simulink model "AutoParking_Parallel_MPC_v2"  (R2021b)
settings: Solver=VariableStepAuto  StartTime=0  StopTime=25  FixedStep=0.01  RelTol=1e-3  AbsTol=1e-6
PreLoadFcn:
  | ParhPoint_Parallel
values from neighbouring files (symbols this model uses):
  dkappa_1 = [dkappa_1,dkappa_1(end)]    [ParhPoint_Parallel.m]    (also in ParhPoint_Parallel1.m)
  dkappa_2 = [dkappa_2,dkappa_2(end)]    [ParhPoint_Parallel.m]    (also in ParhPoint_Parallel1.m)
  dkappa_3 = [dkappa_3,dkappa_3(end)]    [ParhPoint_Parallel.m]    (also in ParhPoint_Parallel1.m)
  dx_1 = [7.49700000000000,7.48700000000000,7.47700000000000,7.46700000000000,7.45700000000000,7.44700000000000,7.43700000000000,7.42700000000000,7.41700000000000,7.40700000000000,7.39700000000000,7.38700000000000,7.37700000000000,7.36700000000000,7.35700000000000,7.34700000000000,7.33700000000000,7.32700000000000,7.31700000000000,7.30700000000000,7.29700000000000,7.28700000000000,7.27700000000000,7.267000 ...(+10617 chars)    [ParhPoint_Parallel1.m]
  dx_2 = xmr01'    [ParhPoint_Parallel.m]    (also in ParhPoint_Parallel1.m = [dx_1(end),1.12])
  dx_3 = [dx_2(end),dx_2(end)]    [ParhPoint_Parallel.m]    (also in ParhPoint_Parallel1.m)
  dy_1 = [1.10000132390871,1.10003103093403,1.10009720896582,1.10019908067609,1.10033587377205,1.10050682098400,1.10071116005326,1.10094813372010,1.10121698971167,1.10151698072983,1.10184736443921,1.10220740345502,1.10259636533104,1.10301352254745,1.10345815249885,1.10392953748209,1.10442696468426,1.10494972617060,1.10549711887234,1.10606844457472,1.10666300990486,1.10728012631967,1.10791911009379,1.108579 ...(+11295 chars)    [ParhPoint_Parallel1.m]
  dy_2 = ymr01'    [ParhPoint_Parallel.m]    (also in ParhPoint_Parallel1.m = [dy_1(end),-1])
  dy_3 = [dy_2(end),dy_2(end)]    [ParhPoint_Parallel.m]    (also in ParhPoint_Parallel1.m)
  dyaw_1 = 0    [ParhPoint_Parallel1.m]
  path_x = [dx_1,dx_2,dx_3]    [ParhPoint_Parallel.m]    (also in ParhPoint_Parallel1.m)
  path_y = [dy_1,dy_2,dy_3]    [ParhPoint_Parallel.m]    (also in ParhPoint_Parallel1.m)
undefined symbols (not defined in the file or in its folder): dyaw_2, dyaw_3
libraries: Solver_SF x1, simulink x1
settings Model: Creator=pmather  LastModifiedBy=Shu
settings SolverCC: AutoScaleAbsTol=off  AlgebraicLoopSolver=TrustRegion
settings DataIOCC: SaveFormat=Array  SignalLoggingSaveFormat=ModelDataLogs  ReturnWorkspaceOutputs=off
settings OptimizationCC: BlockReduction=off  BooleanDataType=off  InitFltsAndDblsToZero=on  LifeSpan=inf
settings DebuggingCC: SaveWithParameterizedLinksMsg=none  UnderspecifiedInitializationDetection=Classic  MergeDetectMultiDrivingBlocksExec=none  SignalResolutionControl=TryResolveAllWithWarning  MultiTaskDSMMsg=warning  MultiTaskCondExecSysMsg=none  SFExecutionAtInitializationDiag=none  SFMachineParentedDataDiag=warning  ArithmeticOperatorsInVariantConditions=warning
settings HardwareCC: ProdBitPerPointer=32  ProdBitPerSizeT=32  ProdBitPerPtrDiffT=32  ProdLargestAtomicFloat=None  ProdIntDivRoundTo=Undefined  ProdEndianess=Unspecified  ProdWordSize=32  ProdHWDeviceType=32-bit Generic  TargetUnknown=on
settings ModelReferenceCC: PropagateSignalLabelsOutOfModel=off
settings SFSimCC: CustomCodeUndefinedFunction=UseInterfaceOnly
settings RTWCC: TemplateMakefile=grt_vc.tmf
settings CodeAppCC: StateflowObjectComments=on
settings GRTTargetCC: TargetLangStandard=C89/C90 (ANSI)  CombineOutputUpdateFcns=off  GRTInterface=on
settings ConfigComp: CovMetricSettings=dw  CovSaveCumulativeToWorkspaceVar=on  CovSaveSingleToWorkspaceVar=on

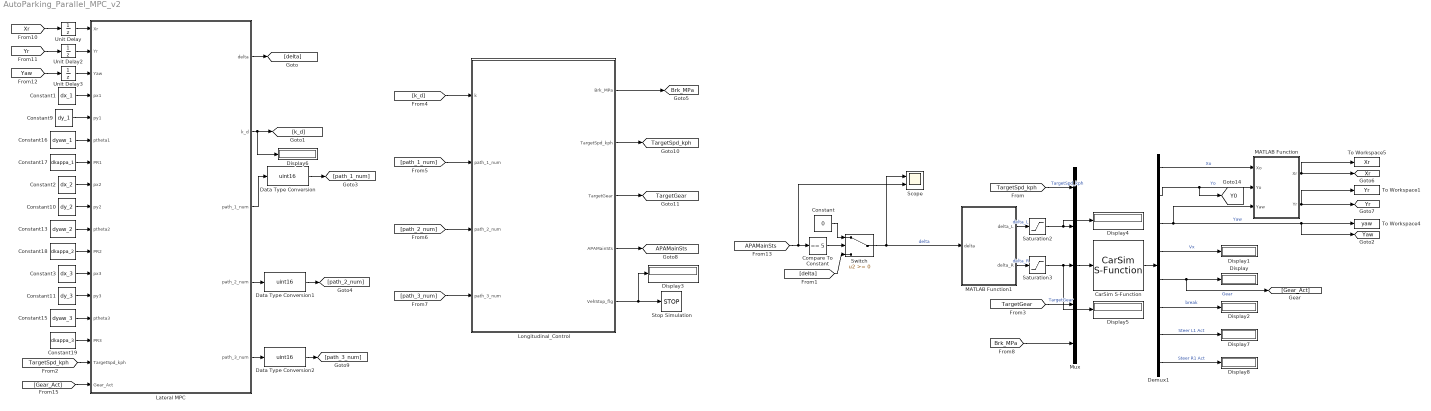
== system AutoParking_Parallel_MPC_v2 ==
  CarSim S-Function : Solver_SF/CarSim S-Function  Priority=1  SIMFILE=simfile.sim
  Compare To Constant : simulink/Logic and Bit Operations/Compare To Constant  relop===  const=5  OutDataTypeStr=boolean
  Constant : Constant  Value=0
  Constant1 : Constant  Value=dx_1
  Constant10 : Constant  Value=dy_2
  Constant11 : Constant  Value=dy_3
  Constant13 : Constant  Value=dyaw_2
  Constant15 : Constant  Value=dyaw_3
  Constant16 : Constant  Value=dyaw_1
  Constant17 : Constant  Value=dkappa_1
  Constant18 : Constant  Value=dkappa_2
  Constant19 : Constant  Value=dkappa_3
  Constant2 : Constant  Value=dx_2
  Constant3 : Constant  Value=dx_3
  Constant9 : Constant  Value=dy_1
  Data Type Conversion : DataTypeConversion  OutDataTypeStr=uint16
  Data Type Conversion1 : DataTypeConversion  OutDataTypeStr=uint16
  Data Type Conversion2 : DataTypeConversion  OutDataTypeStr=uint16
  Demux1 : Demux  Outputs=8
  Display{,1..8} (9 alike) : Display
  Lateral MPC : Subsystem
  Longitudinal_Control : Subsystem
  MATLAB Function : MATLAB Function  TreatAsAtomicUnit=on
  MATLAB Function1 : MATLAB Function  TreatAsAtomicUnit=on
  Mux : Mux  Inputs=5
  Saturation2 : Saturate  UpperLimit=34  LowerLimit=-34
  Saturation3 : Saturate  UpperLimit=34  LowerLimit=-34
  Scope : Scope  NumInputPorts=2
  Stop Simulation : Stop
  Switch : Switch
  To Workspace1 : ToWorkspace  VariableName=Yr  SaveFormat=Timeseries  SampleTime=-1
  To Workspace4 : ToWorkspace  VariableName=yaw  SaveFormat=Timeseries  SampleTime=-1
  To Workspace5 : ToWorkspace  VariableName=Xr  SaveFormat=Timeseries  SampleTime=-1
  Unit Delay : UnitDelay  InitialCondition=1.5  SampleTime=-1  HasFrameUpgradeWarning=on
  Unit Delay2 : UnitDelay  InitialCondition=2.5  SampleTime=-1  HasFrameUpgradeWarning=on
  Unit Delay3 : UnitDelay  SampleTime=-1  HasFrameUpgradeWarning=on
  tag scope: APAMainSts=global, Brk_MPa=global, TargetGear=global, TargetSpd_kph=global, Xr=global, Y0=global, Yaw=global, Yr=global
  wires:
  Mux/1 -> CarSim S-Function/1
  CarSim S-Function/1 -> Demux1/1
  Demux1/1 -> MATLAB Function/1(Xo)  "Xo"
  Demux1/2 -> [Y0], MATLAB Function/2(Yo)  "Yo"
  Demux1/3 -> [Yaw], To Workspace4/1, MATLAB Function/3(Yaw)  "Yaw"
  Demux1/4 -> Display1/1  "Vx"
  MATLAB Function/1(Xr) -> To Workspace5/1, [Xr]
  Longitudinal_Control/1(Brk_MPa) -> [Brk_MPa]
  [Yaw] -> Unit Delay3/1
  [Yr] -> Unit Delay2/1
  [Xr] -> Unit Delay/1
  Unit Delay2/1 -> Lateral MPC/2(Yr)
  Unit Delay/1 -> Lateral MPC/1(Xr)
  Unit Delay3/1 -> Lateral MPC/3(Yaw)
  Constant19/1 -> Lateral MPC/15(PR3)
  Constant18/1 -> Lateral MPC/11(PR2)
  Constant17/1 -> Lateral MPC/7(PR1)
  Constant15/1 -> Lateral MPC/14(ptheta3)
  Constant13/1 -> Lateral MPC/10(ptheta2)
  Constant16/1 -> Lateral MPC/6(ptheta1)
  Constant11/1 -> Lateral MPC/13(py3)
  Constant10/1 -> Lateral MPC/9(py2)
  Constant9/1 -> Lateral MPC/5(py1)
  Constant1/1 -> Lateral MPC/4(px1)
  Constant2/1 -> Lateral MPC/8(px2)
  Constant3/1 -> Lateral MPC/12(px3)
  [Brk_MPa] -> Mux/5
  Demux1/5 -> [Gear_Act], Display/1  "Gear"
  Demux1/6 -> Display2/1  "break"
  Longitudinal_Control/2(TargetSpd_kph) -> [TargetSpd_kph]
  [TargetSpd_kph] -> Mux/1  "TargetSpd_kph"
  Longitudinal_Control/3(TargetGear) -> [TargetGear]
  [TargetGear] -> Mux/4  "TargetGear"
  [TargetSpd_kph] -> Lateral MPC/16(TargetSpd_kph)
  MATLAB Function/2(Yr) -> To Workspace1/1, [Yr]
  Lateral MPC/1(delta) -> [delta]
  Lateral MPC/2(k_d) -> [k_d], Display6/1
  [k_d] -> Longitudinal_Control/1(k)
  [path_2_num] -> Longitudinal_Control/3(path_2_num)
  [path_3_num] -> Longitudinal_Control/4(path_3_num)
  [path_1_num] -> Longitudinal_Control/2(path_1_num)
  Lateral MPC/3(path_1_num) -> Data Type Conversion/1
  Data Type Conversion/1 -> [path_1_num]
  Lateral MPC/4(path_2_num) -> Data Type Conversion1/1
  Data Type Conversion1/1 -> [path_2_num]
  Lateral MPC/5(path_3_num) -> Data Type Conversion2/1
  Data Type Conversion2/1 -> [path_3_num]
  Demux1/7 -> Display7/1  "Steer L1 Act"
  Demux1/8 -> Display8/1  "Steer R1 Act"
  Saturation2/1 -> Display4/1, Mux/2
  Saturation3/1 -> Mux/3, Display5/1
  Longitudinal_Control/4(APAMainSts) -> [APAMainSts]
  Longitudinal_Control/5(VehStop_flg) -> Display3/1, Stop Simulation/1
  [Gear_Act] -> Lateral MPC/17(Gear_Act)
  Switch/1 -> MATLAB Function1/1(delta), Scope/1  "delta"
  MATLAB Function1/1(delta_L) -> Saturation2/1  "delta_L"
  MATLAB Function1/2(delta_R) -> Saturation3/1  "delta_R"
  [APAMainSts] -> Scope/2, Compare To Constant/1
  Compare To Constant/1 -> Switch/2
  Constant/1 -> Switch/1
  [delta] -> Switch/3

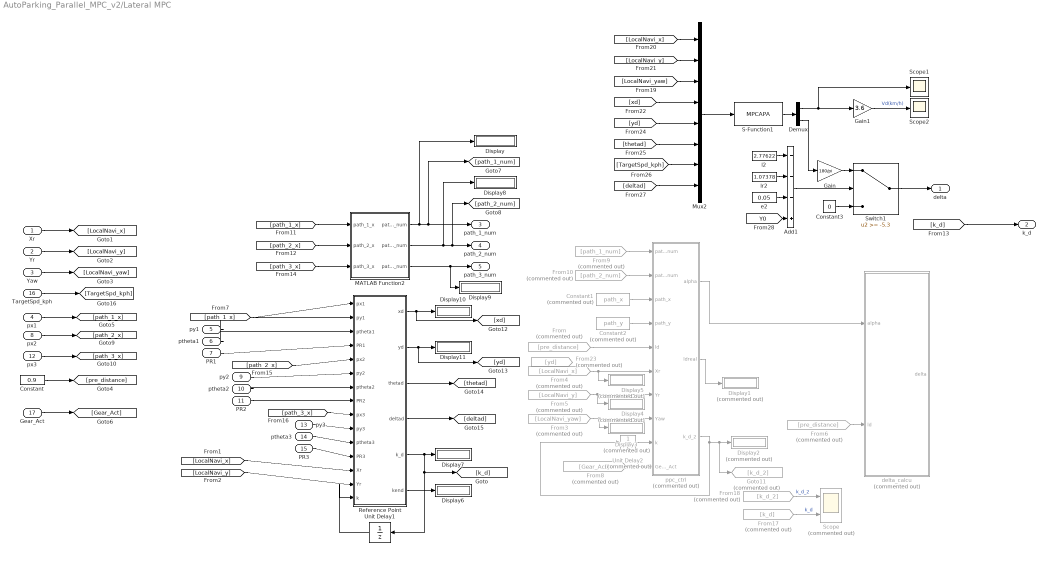
== system AutoParking_Parallel_MPC_v2/Lateral MPC ==
  Xr : Inport
  Yr : Inport  Port=2
  Yaw : Inport  Port=3
  px1 : Inport  Port=4
  py1 : Inport  Port=5
  ptheta1 : Inport  Port=6
  PR1 : Inport  Port=7
  px2 : Inport  Port=8
  py2 : Inport  Port=9
  ptheta2 : Inport  Port=10
  PR2 : Inport  Port=11
  px3 : Inport  Port=12
  py3 : Inport  Port=13
  ptheta3 : Inport  Port=14
  PR3 : Inport  Port=15
  TargetSpd_kph : Inport  Port=16
  Gear_Act : Inport  Port=17
  Add1 : Sum  Inputs=---+
  Constant : Constant  Value=0.9
  Constant1 : Constant  Commented=on  Value=path_x
  Constant2 : Constant  Commented=on  Value=path_y
  Constant3 : Constant  Value=0
  Demux : Demux  Outputs=2
  Display{,6..11} (7 alike) : Display
  Display{1..5} (5 alike) : Display  Commented=on
  From : From  Commented=on  GotoTag=pre_distance
  From10 : From  Commented=on  GotoTag=path_2_num
  From17 : From  Commented=on  GotoTag=k_d
  From18 : From  Commented=on  GotoTag=k_d_2
  From23 : From  Commented=on  GotoTag=yd
  From3 : From  Commented=on  GotoTag=LocalNavi_yaw
  From4 : From  Commented=on  GotoTag=LocalNavi_x
  From5 : From  Commented=on  GotoTag=LocalNavi_y
  From6 : From  Commented=on  GotoTag=pre_distance
  From8 : From  Commented=on  GotoTag=Gear_Act
  From9 : From  Commented=on  GotoTag=path_1_num
  Gain : Gain  Gain=180/pi
  Gain1 : Gain  Gain=3.6
  Goto11 : Goto  Commented=on  GotoTag=k_d_2
  MATLAB Function2 : MATLAB Function  TreatAsAtomicUnit=on
  Mux2 : Mux  Inputs=8
  Reference Point : MATLAB Function  TreatAsAtomicUnit=on
  S-Function1 : S-Function  FunctionName=MPCAPA  SFunctionDeploymentMode=off  EnableBusSupport=off
  Scope : Scope  Commented=on  NumInputPorts=2
  Scope1 : Scope
  Scope2 : Scope
  Switch1 : Switch  Threshold=-5.3
  Unit Delay1 : UnitDelay  InitialCondition=1  SampleTime=-1  HasFrameUpgradeWarning=on
  Unit Delay2 : UnitDelay  Commented=on  InitialCondition=1  SampleTime=-1  HasFrameUpgradeWarning=on
  delta_calcu : MATLAB Function  Commented=on  TreatAsAtomicUnit=on
  e2 : Constant  Value=0.05
  l2 : Constant  Value=2.77622
  lr2 : Constant  Value=1.07378
  ppc_ctrl : MATLAB Function  Commented=on  TreatAsAtomicUnit=on
  delta : Outport
  k_d : Outport  Port=2
  path_1_num : Outport  Port=3
  path_2_num : Outport  Port=4
  path_3_num : Outport  Port=5
  wires:
  Unit Delay1/1 -> Reference Point/15(k)
  Reference Point/5(k_d) -> Display7/1, [k_d], Unit Delay1/1
  py2/1 -> Reference Point/6(py2)
  ptheta2/1 -> Reference Point/7(ptheta2)
  PR2/1 -> Reference Point/8(PR2)
  py3/1 -> Reference Point/10(py3)
  ptheta3/1 -> Reference Point/11(ptheta3)
  PR3/1 -> Reference Point/12(PR3)
  Reference Point/3(thetad) -> [thetad]
  Reference Point/4(deltad) -> [deltad]
  TargetSpd_kph/1 -> [TargetSpd_kph]
  Xr/1 -> [LocalNavi_x]
  Yr/1 -> [LocalNavi_y]
  Yaw/1 -> [LocalNavi_yaw]
  [LocalNavi_x] -> Reference Point/13(Xr)
  [LocalNavi_y] -> Reference Point/14(Yr)
  Constant/1 -> [pre_distance]
  From/1 -> ppc_ctrl/5(ld)
  From5/1 -> Display4/1, ppc_ctrl/7(Yr)
  From4/1 -> Display5/1, ppc_ctrl/6(Xr)
  From3/1 -> Display3/1, ppc_ctrl/8(Yaw)
  ppc_ctrl/1(alpha) -> delta_calcu/1(alpha)
  ppc_ctrl/2(ldreal) -> Display1/1
  ppc_ctrl/3(k_d_2) -> Unit Delay2/1, Goto11/1, Display2/1
  Unit Delay2/1 -> ppc_ctrl/9(k)
  From6/1 -> delta_calcu/2(ld)
  px1/1 -> [path_1_x]
  [path_1_x] -> Reference Point/1(px1)
  [k_d] -> k_d/1
  Reference Point/6(kend) -> Display6/1
  Constant1/1 -> ppc_ctrl/3(path_x)
  Constant2/1 -> ppc_ctrl/4(path_y)
  [path_1_x] -> MATLAB Function2/1(path_1_x)
  px2/1 -> [path_2_x]
  [path_2_x] -> MATLAB Function2/2(path_2_x)
  px3/1 -> [path_3_x]
  [path_3_x] -> MATLAB Function2/3(path_3_x)
  [path_2_x] -> Reference Point/5(px2)
  [path_3_x] -> Reference Point/9(px3)
  MATLAB Function2/1(path_1_num) -> path_1_num/1, [path_1_num], Display/1
  MATLAB Function2/2(path_2_num) -> [path_2_num], path_2_num/1, Display8/1
  MATLAB Function2/3(path_3_num) -> path_3_num/1, Display9/1
  From17/1 -> Scope/2  "k_d"
  From18/1 -> Scope/1  "k_d_2"
  py1/1 -> Reference Point/2(py1)
  ptheta1/1 -> Reference Point/3(ptheta1)
  PR1/1 -> Reference Point/4(PR1)
  Reference Point/1(xd) -> [xd], Display10/1
  Reference Point/2(yd) -> [yd], Display11/1
  Gear_Act/1 -> [Gear_Act]
  From8/1 -> ppc_ctrl/10(Gear_Act)
  From9/1 -> ppc_ctrl/1(path_1_num)
  From10/1 -> ppc_ctrl/2(path_2_num)
  [LocalNavi_yaw] -> Mux2/3
  [LocalNavi_x] -> Mux2/1
  [LocalNavi_y] -> Mux2/2
  [xd] -> Mux2/4
  [yd] -> Mux2/5
  [thetad] -> Mux2/6
  [TargetSpd_kph] -> Mux2/7
  [deltad] -> Mux2/8
  S-Function1/1 -> Demux/1
  l2/1 -> Add1/1
  Gain/1 -> Switch1/1
  Mux2/1 -> S-Function1/1
  Switch1/1 -> delta/1
  Gain1/1 -> Scope2/1  "Vd(km/h)"
  Add1/1 -> Switch1/2
  [Y0] -> Add1/4
  Demux/1 -> Scope1/1, Gain1/1
  Demux/2 -> Gain/1
  lr2/1 -> Add1/2
  Constant3/1 -> Switch1/3
  e2/1 -> Add1/3

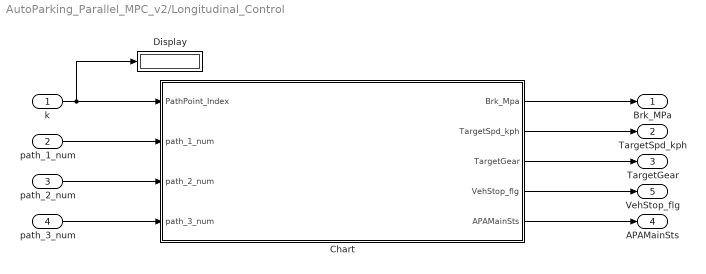
== system AutoParking_Parallel_MPC_v2/Longitudinal_Control ==
  k : Inport
  path_1_num : Inport  Port=2
  path_2_num : Inport  Port=3
  path_3_num : Inport  Port=4
  Chart : Stateflow chart  TreatAsAtomicUnit=on
  Display : Display
  Brk_MPa : Outport
  TargetSpd_kph : Outport  Port=2  VectorParamsAs1DForOutWhenUnconnected=off
  TargetGear : Outport  Port=3  VectorParamsAs1DForOutWhenUnconnected=off
  APAMainSts : Outport  Port=4
  VehStop_flg : Outport  Port=5
  wires:
  k/1 -> Display/1, Chart/1(PathPoint_Index)
  Chart/1(Brk_Mpa) -> Brk_MPa/1
  Chart/2(TargetSpd_kph) -> TargetSpd_kph/1
  Chart/3(TargetGear) -> TargetGear/1
  path_1_num/1 -> Chart/2(path_1_num)
  path_2_num/1 -> Chart/3(path_2_num)
  path_3_num/1 -> Chart/4(path_3_num)
  Chart/4(VehStop_flg) -> VehStop_flg/1
  Chart/5(APAMainSts) -> APAMainSts/1

== matlab function AutoParking_Parallel_MPC_v2/MATLAB Function ==
  data: Xo input; Xr output; Yo input; Yaw input; Yr output
%% 将质心的坐标转换为后轴中心坐标
function [Xr,Yr] = fcn(Xo,Yo,Yaw)
l=2.77622;%轴距
Xr=Xo-l*cos(Yaw/180*pi);
Yr=Yo-l*sin(Yaw/180*pi);

== matlab function AutoParking_Parallel_MPC_v2/Lateral MPC/delta_calcu ==
  data: alpha input; delta output; ld input
function delta = fcn(alpha,ld)
L=2.66;
delta=atan(2*L*sin(alpha)/ld);

== matlab function AutoParking_Parallel_MPC_v2/Lateral MPC/ppc_ctrl ==
  data: path_1_num input; path_2_num input; path_x input; path_y input; ld input; Xr input; Yr input; alpha output; Yaw input; k input; ldreal output; k_d_2 output; Gear_Act input
function [alpha,ldreal,k_d_2] = fcn(path_1_num,path_2_num,path_x,path_y,ld,Xr,Yr,Yaw,k,Gear_Act)

%初始化最小误差和参考点索引
emin=0.9;
k_d_2=k;

path_length = 0;

if Gear_Act==-1
    path_length = path_1_num;
end

if Gear_Act==1
    path_length = path_1_num+path_2_num;
end

%确定搜索参考点范围
if k+30>=path_length
    kend=path_length;
else
    kend=k+30;
end

%搜索参考点
for i=k:kend
   e=abs(sqrt((Xr-path_x(i))^2+(Yr-path_y(i))^2)-ld);
   if e<emin
       emin=e;
       k_d_2=i;
   end
end

ldreal=sqrt((Xr-path_x(k_d_2))^2+(Yr-path_y(k_d_2))^2);

%计算角度偏差
Yaw=mod(Yaw/180*pi,2*pi);%车辆横摆角转化为0~2*pi的弧度
theta=atan2((path_y(k_d_2)-Yr),(path_x(k_d_2)-Xr));%-pi~pi的弧度
%转化为0~2*pi的弧度
if theta<0
    theta=theta+2*pi;
end

alpha=theta-Yaw;

== stateflow chart AutoParking_Parallel_MPC_v2/Longitudinal_Control/Chart ==
  state Path_0_Start
    en:
    APAMainSts=0;
    VehStop_flg=0;
    Brk_Mpa = 0;
    TargetSpd_kph = 0;
    TargetGear = 0;
    Counter = 0;
    du:
    Counter++;
  state Path_1_Start
    en:
    APAMainSts=2;
    Brk_Mpa = 0;
    state Path_2_Gear
      en:
      TargetGear = -1;
      Counter = 0;
      du:
      Counter++;
    state Path_2_Speed
      en:
      TargetSpd_kph = -3;
    state Path_2_Speed1
      en:
      TargetSpd_kph = -1;
    state Path_2_Speed2
      en:
      TargetSpd_kph = -0.5;
      Brk_Mpa = 0.2;
    Path_1_Start.Path_2_Gear -> Path_1_Start.Path_2_Speed : [Counter>1000]
    Path_1_Start.Path_2_Speed -> Path_1_Start.Path_2_Speed1 : [PathPoint_Index>(path_1_num-70)]
    Path_1_Start.Path_2_Speed1 -> Path_1_Start.Path_2_Speed2 : [PathPoint_Index > (path_1_num-35)]
  state Path_1_End
    en:
    Brk_Mpa = 5;
    Counter = 0;
    TargetSpd_kph = 0;
    du:
    Counter++;
  state Steer_Reset1
    en:
    Brk_Mpa = 5;
    APAMainSts=3;
    Counter = 0;
    Brk_Mpa = 0;
    TargetGear = 0;
    TargetSpd_kph = 0;
    du:
    Counter++;
  state Path_2_Start
    state Path_2_Gear
      en:
      Brk_Mpa = 0;
      TargetGear = 1;
      Counter = 0;
      du:
      Counter++;
    state Path_2_Speed
      en:
      Brk_Mpa = 0;
      TargetSpd_kph = 2;
    state Path_2_Speed1
      en:
      TargetSpd_kph = 1;
    state Path_2_Speed2
      en:
      TargetSpd_kph = 0.5;
    Path_2_Start.Path_2_Gear -> Path_2_Start.Path_2_Speed : [Counter>=1500]
    Path_2_Start.Path_2_Speed -> Path_2_Start.Path_2_Speed1 : [PathPoint_Index>path_1_num+path_2_num-70]
    Path_2_Start.Path_2_Speed1 -> Path_2_Start.Path_2_Speed2 : [PathPoint_Index>path_1_num+path_2_num-35]
  note: function y = fcn(u1,u3)
      |
      | if u1>=311 && u1<=315    %if (u1>=311 && u1<=315) || u2<-5.3
      |     y=10;
      | elseif u1>=468 && u1<=472
      |     y=15;
      | elseif u1>=1255 && u1<=1261
      |     y=10;
      | else
      |     y=u3;
      | end
  state Path_2_Brake
    en:
    Counter = 0;
    TargetSpd_kph = 0;
    Brk_Mpa = 5;
    du:
    Counter++;
  state Path_3_Start [commented out]
    en:
    Brk_Mpa = 0;
    state Path_2_Gear [commented out]
      en:
      TargetGear = -1;
      Counter = 0;
      du:
      Counter++;
    state Path_2_Speed [commented out]
      en:
      TargetSpd_kph = -2;
    Path_3_Start.Path_2_Gear -> Path_3_Start.Path_2_Speed [commented out] : [Counter>=1500]
  state Steer_Reset
    en:
    APAMainSts=3;
    Counter = 0;
    Brk_Mpa = 0;
    TargetGear = 0;
    TargetSpd_kph = 0;
    du:
    Counter++;
  state Path_3_Brake [commented out]
    en:
    Brk_Mpa = 10;
    Counter = 0;
    TargetSpd_kph = 0;
    du:
    Counter++;
  state Wait
    en:
    APAMainSts=5;
    Brk_Mpa = 5;
    VehStop_flg=0;
    Counter = 0;
    du:
    Counter++;
  state End
    en:
    VehStop_flg=1;
  (default) -> Path_0_Start
  Path_0_Start -> Path_1_Start.Path_2_Gear : [Counter>1000]
  Path_1_Start -> Path_1_End : [PathPoint_Index >= path_1_num-2]
  Path_1_End -> Steer_Reset1 : [Counter >= 1500]
  Steer_Reset1 -> Path_2_Start.Path_2_Gear : [Counter>=100]
  Path_2_Start.Path_2_Speed2 -> Path_2_Brake : [PathPoint_Index > (path_1_num+path_2_num)]
  Path_2_Brake -> (junction 90) : [Counter >= 100]
  (junction 90) -> (junction 80)
  Path_2_Brake -> Path_3_Start.Path_2_Gear [commented out] : [Counter >= 1500&&PathPoint_Index > path_1_num+path_2_num]
  (junction 80) -> Steer_Reset
  Path_3_Start.Path_2_Speed -> Path_3_Brake [commented out] : [PathPoint_Index > (path_1_num+path_2_num+path_3_num-25)]
  Path_3_Brake -> Wait [commented out] : [Counter>1500]
  Steer_Reset -> (junction 82) : [Counter>2100]
  (junction 82) -> Wait
  Wait -> End : [Counter>100]
  data: PathPoint_Index input; Counter local uint16; Brk_Mpa output double; TargetSpd_kph output double; TargetGear output; VehStop_flg output boolean; path_1_num input uint16; path_2_num input uint16; path_3_num input uint16; APAMainSts output uint8

== matlab function AutoParking_Parallel_MPC_v2/Lateral MPC/Reference Point ==
  data: px1 input; py1 input; ptheta1 input; PR1 input; px2 input; py2 input; ptheta2 input; PR2 input; px3 input; py3 input; ptheta3 input; PR3 input; xd output; yd output; thetad output; deltad output; Xr input; Yr input; k input; k_d output; kend output
function [xd,yd,thetad,deltad,k_d,kend] = fcn(px1,py1,ptheta1,PR1,px2,py2,ptheta2,PR2,px3,py3,ptheta3,PR3,Xr,Yr,k)
l=2.66; % D级车SUV
e_min=1;
k_d=k; % k是k_d上一周期的数据,初始值为0,即k_d_delay; k_d是当前位置的序号;
kend=k_d+50;
%%%%%%%%%%%%%%%%%%%%%%%%%%%%%%%%%%%%%%%%%%%%%%%%%%%%%%%
if k_d<length(px1)
    if kend>=length(px1)
        kend=length(px1);
    end
    for i=k:kend
        e=sqrt((Xr-px1(i))^2+(Yr-py1(i))^2);
        if e<e_min
            e_min=e;
            k_d=i;
        end
    end
    xd=px1(k_d);
    yd=py1(k_d);
    thetad=ptheta1(k_d);
    deltad=-atan(l*PR1(k_d));
%%%%%%%%%%%%%%%%%%%%%%%%%%%%%%%%%%%%%%%%%%%%%%%%%%%%%%%
elseif k==length(px1)
    k_d=length(px1)+1;
    xd=px2(k_d-length(px1));
    yd=py2(k_d-length(px1));
    thetad=ptheta2(k_d-length(px1));
    deltad=atan(l*PR2(k_d-length(px1)));
    
%%%%%%%%%%%%%%%%%%%%%%%%%%%%%%%%%%%%%%%%%%%%%%%%%%%%%%
elseif k<length(px1)+length(px2)
    if kend>=length(px1)+length(px2)
        kend=length(px1)+length(px2);
    end
    for i=k:kend
        e=sqrt((Xr-px2(i-length(px1)))^2+(Yr-py2(i-length(px1)))^2);
        if e<e_min
            e_min=e;
            k_d=i;
        end
    end
    xd=px2(k_d-length(px1));
    yd=py2(k_d-length(px1));
    thetad=ptheta2(k_d-length(px1));
    deltad=atan(l*PR2(k_d-length(px1)));
%     vd=2;
%     gear=1;
%%%%%%%%%%%%%%%%%%%%%%%%%%%%%%%%%%%%%%%%%%%%%%%%%%%%%%%
elseif k==length(px1)+length(px2)
    k_d=length(px1)+length(px2)+1;
    xd=px3(k_d-length(px1)-length(px2));
    yd=py3(k_d-length(px1)-length(px2));
    thetad=ptheta3(k_d-length(px1)-length(px2));
    deltad=-atan(l*PR3(k_d-length(px1)-length(px2)));
%%%%%%%%%%%%%%%%%%%%%%%%%%%%%%%%%%%%%%%%%%%%%%%%%%%%%%%
else
    if kend>=length(px1)+length(px2)+length(px3)
        kend=length(px1)+length(px2)+length(px3);
    end
    for i=k:kend
        e=sqrt((Xr-px3(i-length(px1)-length(px2)))^2+(Yr-py3(i-length(px1)-length(px2)))^2);
        if e<e_min
            e_min=e;
            k_d=i;
        end
    end
    xd=px3(k_d-length(px1)-length(px2));
    yd=py3(k_d-length(px1)-length(px2));
    thetad=ptheta3(k_d-length(px1)-length(px2));
    deltad=-atan(l*PR3(k_d-length(px1)-length(px2)));
end

== matlab function AutoParking_Parallel_MPC_v2/Lateral MPC/MATLAB Function2 ==
  data: path_1_x input; path_1_num output; path_2_x input; path_3_x input; path_2_num output; path_3_num output
function[path_1_num,path_2_num,path_3_num] = fcn(path_1_x,path_2_x,path_3_x)

path_1_num = length(path_1_x);
path_2_num = length(path_2_x);
path_3_num = length(path_3_x);


end

== matlab function AutoParking_Parallel_MPC_v2/MATLAB Function1 ==
  data: delta input; delta_L output; delta_R output
function [delta_L,delta_R] = fcn(delta)
% l=2.77622;
% L1=1.545;
l=2.66;
L1=1.845;
tan_delta_L=1/(1/(tan(delta/180*pi))-(L1/2)/l);
tan_delta_R=1/(1/(tan(delta/180*pi))+(L1/2)/l);
delta_L=atan(tan_delta_L)/pi*180;
delta_R=atan(tan_delta_R)/pi*180;
